simulink model "umv"  (R2019b)
settings: Solver=VariableStepAuto  StartTime=0.0  StopTime=10.0  RelTol=1e-3
InitFcn:
  | umvInit;
undefined symbols (not defined in the file): A, B, C, D, G, H, stateInit, Ts
settings Model: Creator=louis  LastModifiedBy=louis

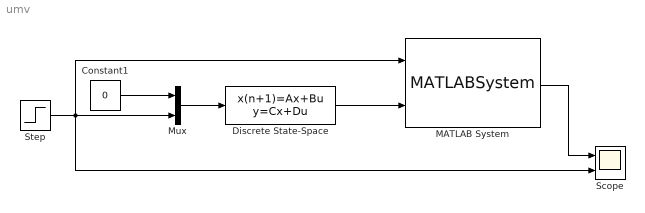
== system umv ==
  Constant1 : Constant  Value=0  SampleTime=Ts
  Discrete State-Space : DiscreteStateSpace  A=A  B=[B H]  C=C  D=[D G]  InitialCondition=stateInit  SampleTime=Ts
  MATLAB System : MATLABSystem  System=UMV  ModelSourceChoice=Individual matrices  AMat=A  BMat=B  HMat=H  CMat=C  DMat=D  GMat=G  NxUserDefined=1  NuUserDefined=1  NeUserDefined=1  NyUserDefined=1  Ts=Ts  xInit=stateInitUmv  PInit=PInit  isQTimeInvariant=on  QMat=Q  isRTimeInvariant=on  RMat=R  hasKnownInput=on  showEstimatedState=off  showEstimatedInputs=on  showEstimatedOutput=off  showStateCovariance=off
      mask Type: UMV
      mask Display:
      | disp(['Unbiased' char(10) 'Minimum' char(10) 'Variance' char(10) 'Filter']);
      | port_label('input',1,'u');
      | port_label('input',2,'y');
      | port_label('output',1,'ehat');
  Mux : Mux  Inputs=2
  Scope : Scope  NumInputPorts=2
  Step : Step  After=10  SampleTime=Ts
  wires:
  Discrete State-Space/1 -> MATLAB System/2
  Mux/1 -> Discrete State-Space/1
  Step/1 -> Scope/2, MATLAB System/1, Mux/2
  Constant1/1 -> Mux/1
  MATLAB System/1 -> Scope/1
